simulink model "Open_Closed_Loop"  (R2022b)
settings: Solver=VariableStepAuto  StartTime=0.0  StopTime=10.0  RelTol=1e-3
settings Model: Creator=MAAM  LastModifiedBy=MAAM

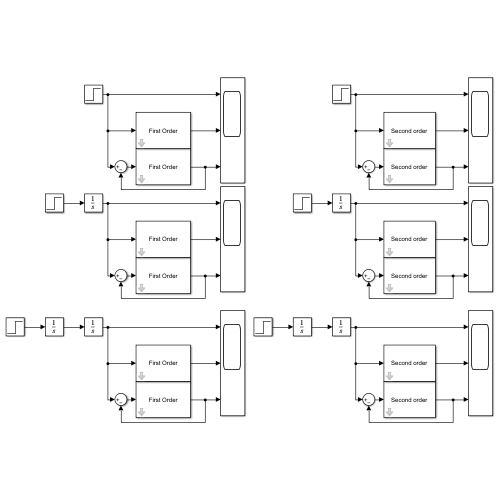
[thumbnail: Simulink's stored preview of the top-level diagram]
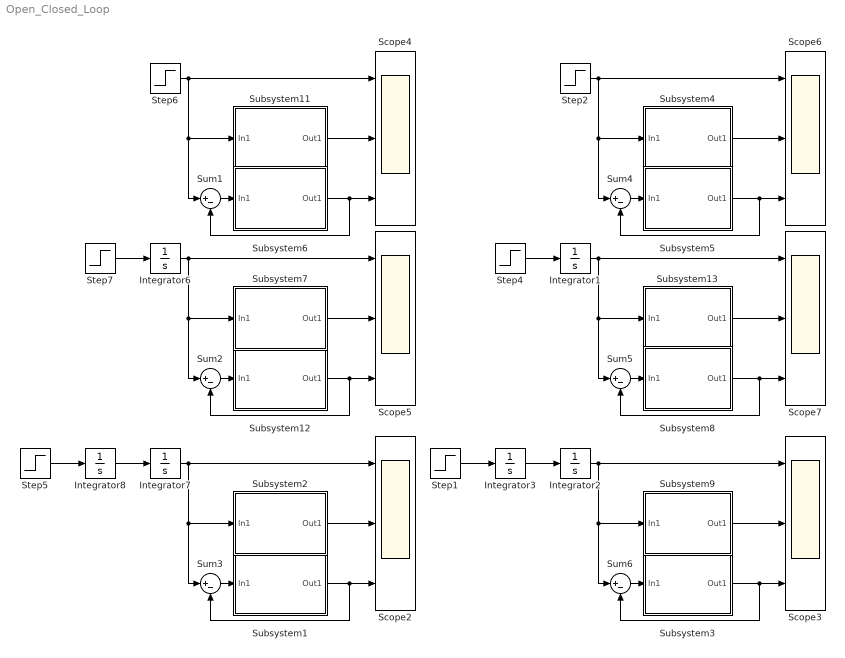
== system Open_Closed_Loop ==
  Integrator{1..3,6..8} (6 alike) : Integrator
  Scope{2..7} (6 alike) : Scope  NumInputPorts=3
  Step{1..2,4..7} (6 alike) : Step  SampleTime=0
  Subsystem1 : Subsystem  mask{T=0.25, K=1}
      mask prompts: T "Time Constant "T""; K "Gain "K""
      mask Display: fprintf("First Order");
  Subsystem11 : Subsystem  mask{T=0.25, K=1}
      mask prompts: T "Time Constant "T""; K "Gain "K""
      mask Display: fprintf("First Order");
  Subsystem12 : Subsystem  mask{T=0.25, K=1}
      mask prompts: T "Time Constant "T""; K "Gain "K""
      mask Display: fprintf("First Order");
  Subsystem13 : Subsystem  mask{W_n=1, Z=1}
      mask prompts: W_n "Natural frequency "\omega_n""; Z "Damping Constant "\zeta""
      mask Display: fprintf("Second order");
  Subsystem2 : Subsystem  mask{T=0.25, K=1}
      mask prompts: T "Time Constant "T""; K "Gain "K""
      mask Display: fprintf("First Order");
  Subsystem3 : Subsystem  mask{W_n=1, Z=1}
      mask prompts: W_n "Natural frequency "\omega_n""; Z "Damping Constant "\zeta""
      mask Display: fprintf("Second order");
  Subsystem4 : Subsystem  mask{W_n=1, Z=1}
      mask prompts: W_n "Natural frequency "\omega_n""; Z "Damping Constant "\zeta""
      mask Display: fprintf("Second order");
  Subsystem5 : Subsystem  mask{W_n=1, Z=1}
      mask prompts: W_n "Natural frequency "\omega_n""; Z "Damping Constant "\zeta""
      mask Display: fprintf("Second order");
  Subsystem6 : Subsystem  mask{T=0.25, K=1}
      mask prompts: T "Time Constant "T""; K "Gain "K""
      mask Display: fprintf("First Order");
  Subsystem7 : Subsystem  mask{T=0.25, K=1}
      mask prompts: T "Time Constant "T""; K "Gain "K""
      mask Display: fprintf("First Order");
  Subsystem8 : Subsystem  mask{W_n=1, Z=1}
      mask prompts: W_n "Natural frequency "\omega_n""; Z "Damping Constant "\zeta""
      mask Display: fprintf("Second order");
  Subsystem9 : Subsystem  mask{W_n=1, Z=1}
      mask prompts: W_n "Natural frequency "\omega_n""; Z "Damping Constant "\zeta""
      mask Display: fprintf("Second order");
  Sum{1..6} (6 alike) : Sum  Inputs=|+-
  wires:
  Integrator8/1 -> Integrator7/1
  Step5/1 -> Integrator8/1
  Step7/1 -> Integrator6/1
  Subsystem6/1(Out1) -> Sum1/2, Scope4/3
  Step6/1 -> Sum1/1, Subsystem11/1(In1), Scope4/1
  Sum1/1 -> Subsystem6/1(In1)
  Subsystem11/1(Out1) -> Scope4/2
  Subsystem7/1(Out1) -> Scope5/2
  Sum2/1 -> Subsystem12/1(In1)
  Integrator6/1 -> Scope5/1, Subsystem7/1(In1), Sum2/1
  Subsystem12/1(Out1) -> Scope5/3, Sum2/2
  Subsystem1/1(Out1) -> Sum3/2, Scope2/3
  Integrator7/1 -> Sum3/1, Subsystem2/1(In1), Scope2/1
  Sum3/1 -> Subsystem1/1(In1)
  Subsystem2/1(Out1) -> Scope2/2
  Subsystem9/1(Out1) -> Scope3/2
  Sum6/1 -> Subsystem3/1(In1)
  Integrator2/1 -> Scope3/1, Subsystem9/1(In1), Sum6/1
  Subsystem3/1(Out1) -> Scope3/3, Sum6/2
  Subsystem8/1(Out1) -> Sum5/2, Scope7/3
  Integrator1/1 -> Subsystem13/1(In1), Sum5/1, Scope7/1
  Sum5/1 -> Subsystem8/1(In1)
  Subsystem13/1(Out1) -> Scope7/2
  Subsystem4/1(Out1) -> Scope6/2
  Sum4/1 -> Subsystem5/1(In1)
  Step2/1 -> Scope6/1, Subsystem4/1(In1), Sum4/1
  Subsystem5/1(Out1) -> Scope6/3, Sum4/2
  Step4/1 -> Integrator1/1
  Step1/1 -> Integrator3/1
  Integrator3/1 -> Integrator2/1

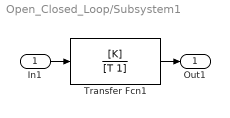
== system Open_Closed_Loop/Subsystem1 ==
  In1 : Inport
  Transfer Fcn1 : TransferFcn  Numerator=[K]  Denominator=[T 1]
  Out1 : Outport
  wires:
  In1/1 -> Transfer Fcn1/1
  Transfer Fcn1/1 -> Out1/1

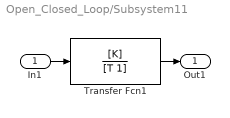
== system Open_Closed_Loop/Subsystem11 ==
  In1 : Inport
  Transfer Fcn1 : TransferFcn  Numerator=[K]  Denominator=[T 1]
  Out1 : Outport
  wires:
  In1/1 -> Transfer Fcn1/1
  Transfer Fcn1/1 -> Out1/1

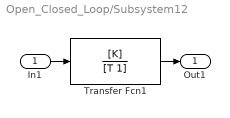
== system Open_Closed_Loop/Subsystem12 ==
  In1 : Inport
  Transfer Fcn1 : TransferFcn  Numerator=[K]  Denominator=[T 1]
  Out1 : Outport
  wires:
  Transfer Fcn1/1 -> Out1/1
  In1/1 -> Transfer Fcn1/1

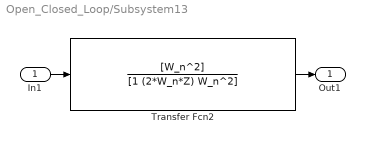
== system Open_Closed_Loop/Subsystem13 ==
  In1 : Inport
  Transfer Fcn2 : TransferFcn  Numerator=[W_n^2]  Denominator=[1 (2*W_n*Z) W_n^2]
  Out1 : Outport
  wires:
  Transfer Fcn2/1 -> Out1/1
  In1/1 -> Transfer Fcn2/1

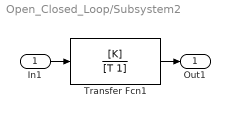
== system Open_Closed_Loop/Subsystem2 ==
  In1 : Inport
  Transfer Fcn1 : TransferFcn  Numerator=[K]  Denominator=[T 1]
  Out1 : Outport
  wires:
  In1/1 -> Transfer Fcn1/1
  Transfer Fcn1/1 -> Out1/1

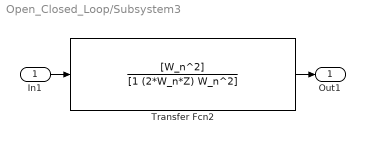
== system Open_Closed_Loop/Subsystem3 ==
  In1 : Inport
  Transfer Fcn2 : TransferFcn  Numerator=[W_n^2]  Denominator=[1 (2*W_n*Z) W_n^2]
  Out1 : Outport
  wires:
  In1/1 -> Transfer Fcn2/1
  Transfer Fcn2/1 -> Out1/1

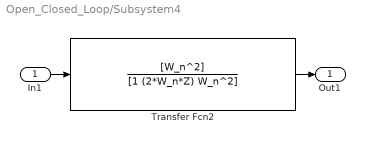
== system Open_Closed_Loop/Subsystem4 ==
  In1 : Inport
  Transfer Fcn2 : TransferFcn  Numerator=[W_n^2]  Denominator=[1 (2*W_n*Z) W_n^2]
  Out1 : Outport
  wires:
  In1/1 -> Transfer Fcn2/1
  Transfer Fcn2/1 -> Out1/1

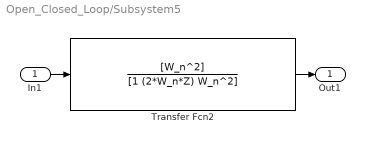
== system Open_Closed_Loop/Subsystem5 ==
  In1 : Inport
  Transfer Fcn2 : TransferFcn  Numerator=[W_n^2]  Denominator=[1 (2*W_n*Z) W_n^2]
  Out1 : Outport
  wires:
  Transfer Fcn2/1 -> Out1/1
  In1/1 -> Transfer Fcn2/1

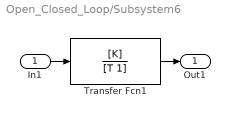
== system Open_Closed_Loop/Subsystem6 ==
  In1 : Inport
  Transfer Fcn1 : TransferFcn  Numerator=[K]  Denominator=[T 1]
  Out1 : Outport
  wires:
  In1/1 -> Transfer Fcn1/1
  Transfer Fcn1/1 -> Out1/1

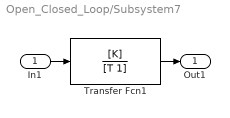
== system Open_Closed_Loop/Subsystem7 ==
  In1 : Inport
  Transfer Fcn1 : TransferFcn  Numerator=[K]  Denominator=[T 1]
  Out1 : Outport
  wires:
  Transfer Fcn1/1 -> Out1/1
  In1/1 -> Transfer Fcn1/1

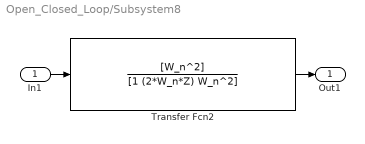
== system Open_Closed_Loop/Subsystem8 ==
  In1 : Inport
  Transfer Fcn2 : TransferFcn  Numerator=[W_n^2]  Denominator=[1 (2*W_n*Z) W_n^2]
  Out1 : Outport
  wires:
  In1/1 -> Transfer Fcn2/1
  Transfer Fcn2/1 -> Out1/1

== system Open_Closed_Loop/Subsystem9 ==
  In1 : Inport
  Transfer Fcn2 : TransferFcn  Numerator=[W_n^2]  Denominator=[1 (2*W_n*Z) W_n^2]
  Out1 : Outport
  wires:
  Transfer Fcn2/1 -> Out1/1
  In1/1 -> Transfer Fcn2/1
